simulink model "ccc_core"  (Simulink 7.4)
settings: Solver=ode45  StartTime=0.0  StopTime=10000  RelTol=1e-3
libraries: xbsIndex_r4 x236, cfa_library x64, casper_library_misc x7
(part 1 of 5)
settings Model: Creator=Administrator  LastModifiedBy=rprimian
settings OptimizationCC: InitFltsAndDblsToZero=on

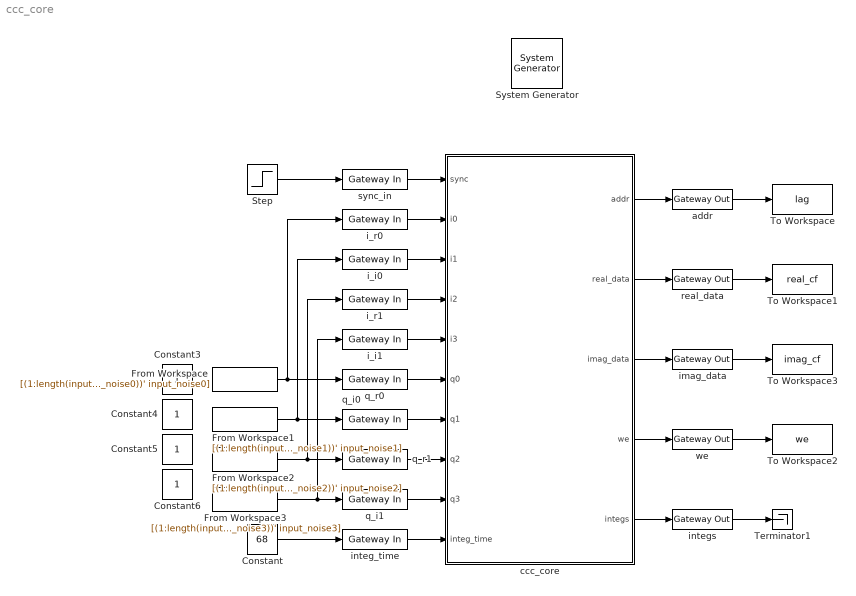
== system ccc_core ==
  " System Generator" : xbsIndex_r4/ System Generator  Tag=genX  SystemSampleTime=-1  xilinxfamily=virtex2p  part=xc2vp50  speed=-7  package=ff1152  synthesis_tool=XST  clock_wrapper=Clock Enables  directory=./correlator_core  testbench=off  simulink_period=1  sysclk_period=100  dcm_input_clock_period=100  incr_netlist=off  trim_vbits=Everywhere in SubSystem  dbl_ovrd=According to Block Masks  core_generation=According to Block Masks  run_coregen=off  deprecated_control=off  eval_field=0  block_type=sysgen
      settings: block_version=10.1.3
  Constant : Constant  Value=68  OutDataType=sfix(16)  OutScaling=2^0
  Constant{3..6} (4 alike) : Constant  OutDataType=sfix(16)  OutScaling=2^0
  From Workspace : FromWorkspace  VariableName=[(1:length(input_noise0))' input_noise0]  SampleTime=1  Interpolate=off  OutputAfterFinalValue=Setting to zero
  From Workspace1 : FromWorkspace  VariableName=[(1:length(input_noise1))' input_noise1]  SampleTime=1  Interpolate=off  OutputAfterFinalValue=Setting to zero
  From Workspace2 : FromWorkspace  VariableName=[(1:length(input_noise2))' input_noise2]  SampleTime=1  Interpolate=off  OutputAfterFinalValue=Setting to zero
  From Workspace3 : FromWorkspace  VariableName=[(1:length(input_noise3))' input_noise3]  SampleTime=1  Interpolate=off  OutputAfterFinalValue=Setting to zero
  Step : Step  Time=100  SampleTime=0
  Terminator1 : Terminator
  To Workspace : ToWorkspace  VariableName=lag  SampleTime=-1  SaveFormat=Array
  To Workspace1 : ToWorkspace  VariableName=real_cf  SampleTime=-1  SaveFormat=Array
  To Workspace2 : ToWorkspace  VariableName=we  SampleTime=-1  SaveFormat=Array
  To Workspace3 : ToWorkspace  VariableName=imag_cf  SampleTime=-1  SaveFormat=Array
  addr : xbsIndex_r4/Gateway Out  hdl_port=on  timing_constraint=None  locs_specified=off  LOCs={}  block_type=gatewayout
      settings: infoedit="Gateway out block.  Converts Xilinx fixed point inputs into ouputs of type Simulink integer, double, or fixed point.<P><P>Hardware notes:  In hardware these blocks become top level output ports or are discarded, depending on how they are configured."  block_version=10.1.3
  ccc_core : Subsystem
  i_i0 : xbsIndex_r4/Gateway In  arith_type=Unsigned  n_bits=2  bin_pt=0  quantization=Truncate  overflow=Wrap  period=1  dbl_ovrd=off  timing_constraint=None  locs_specified=off  LOCs={}  hdl_port=on  block_type=gatewayin
      settings: infoedit="Gateway in block.  Converts inputs of type Simulink integer, double and fixed point to  Xilinx fixed point type.<br><br>Hardware notes:  In hardware these blocks become top level input ports."  block_version=10.1.3
  i_i1 : xbsIndex_r4/Gateway In  arith_type=Unsigned  n_bits=2  bin_pt=0  quantization=Truncate  overflow=Wrap  period=1  dbl_ovrd=off  timing_constraint=None  locs_specified=off  LOCs={}  hdl_port=on  block_type=gatewayin
      settings: infoedit="Gateway in block.  Converts inputs of type Simulink integer, double and fixed point to  Xilinx fixed point type.<br><br>Hardware notes:  In hardware these blocks become top level input ports."  block_version=10.1.3
  i_r0 : xbsIndex_r4/Gateway In  arith_type=Unsigned  n_bits=2  bin_pt=0  quantization=Truncate  overflow=Flag as error  period=1  dbl_ovrd=off  timing_constraint=None  locs_specified=off  LOCs={}  hdl_port=on  block_type=gatewayin
      settings: infoedit="Gateway in block.  Converts inputs of type Simulink integer, double and fixed point to  Xilinx fixed point type.<br><br>Hardware notes:  In hardware these blocks become top level input ports."  block_version=10.1.3
  i_r1 : xbsIndex_r4/Gateway In  arith_type=Unsigned  n_bits=2  bin_pt=0  quantization=Truncate  overflow=Wrap  period=1  dbl_ovrd=off  timing_constraint=None  locs_specified=off  LOCs={}  hdl_port=on  block_type=gatewayin
      settings: infoedit="Gateway in block.  Converts inputs of type Simulink integer, double and fixed point to  Xilinx fixed point type.<br><br>Hardware notes:  In hardware these blocks become top level input ports."  block_version=10.1.3
  imag_data : xbsIndex_r4/Gateway Out  hdl_port=on  timing_constraint=None  locs_specified=off  LOCs={}  block_type=gatewayout
      settings: infoedit="Gateway out block.  Converts Xilinx fixed point inputs into ouputs of type Simulink integer, double, or fixed point.<P><P>Hardware notes:  In hardware these blocks become top level output ports or are discarded, depending on how they are configured."  block_version=10.1.3
  integ_time : xbsIndex_r4/Gateway In  arith_type=Unsigned  n_bits=32  bin_pt=0  quantization=Truncate  overflow=Wrap  period=1  dbl_ovrd=off  timing_constraint=None  locs_specified=off  LOCs={}  hdl_port=on  block_type=gatewayin
      settings: infoedit="Gateway in block.  Converts inputs of type Simulink integer, double and fixed point to  Xilinx fixed point type.<P><P>Hardware notes:  In hardware these blocks become top level input ports."  block_version=10.1.3
  integs : xbsIndex_r4/Gateway Out  hdl_port=on  timing_constraint=None  locs_specified=off  LOCs={}  block_type=gatewayout
      settings: infoedit="Gateway out block.  Converts Xilinx fixed point inputs into ouputs of type Simulink integer, double, or fixed point.<P><P>Hardware notes:  In hardware these blocks become top level output ports or are discarded, depending on how they are configured."  block_version=10.1.3
  q_i0 : xbsIndex_r4/Gateway In  arith_type=Unsigned  n_bits=2  bin_pt=0  quantization=Truncate  overflow=Wrap  period=1  dbl_ovrd=off  timing_constraint=None  locs_specified=off  LOCs={}  hdl_port=on  block_type=gatewayin
      settings: infoedit="Gateway in block.  Converts inputs of type Simulink integer, double and fixed point to  Xilinx fixed point type.<br><br>Hardware notes:  In hardware these blocks become top level input ports."  block_version=10.1.3
  q_i1 : xbsIndex_r4/Gateway In  arith_type=Unsigned  n_bits=2  bin_pt=0  quantization=Truncate  overflow=Wrap  period=1  dbl_ovrd=off  timing_constraint=None  locs_specified=off  LOCs={}  hdl_port=on  block_type=gatewayin
      settings: infoedit="Gateway in block.  Converts inputs of type Simulink integer, double and fixed point to  Xilinx fixed point type.<br><br>Hardware notes:  In hardware these blocks become top level input ports."  block_version=10.1.3
  q_r0 : xbsIndex_r4/Gateway In  arith_type=Unsigned  n_bits=2  bin_pt=0  quantization=Truncate  overflow=Wrap  period=1  dbl_ovrd=off  timing_constraint=None  locs_specified=off  LOCs={}  hdl_port=on  block_type=gatewayin
      settings: infoedit="Gateway in block.  Converts inputs of type Simulink integer, double and fixed point to  Xilinx fixed point type.<br><br>Hardware notes:  In hardware these blocks become top level input ports."  block_version=10.1.3
  q_r1 : xbsIndex_r4/Gateway In  arith_type=Unsigned  n_bits=2  bin_pt=0  quantization=Truncate  overflow=Wrap  period=1  dbl_ovrd=off  timing_constraint=None  locs_specified=off  LOCs={}  hdl_port=on  block_type=gatewayin
      settings: infoedit="Gateway in block.  Converts inputs of type Simulink integer, double and fixed point to  Xilinx fixed point type.<br><br>Hardware notes:  In hardware these blocks become top level input ports."  block_version=10.1.3
  real_data : xbsIndex_r4/Gateway Out  hdl_port=on  timing_constraint=None  locs_specified=off  LOCs={}  block_type=gatewayout
      settings: infoedit="Gateway out block.  Converts Xilinx fixed point inputs into ouputs of type Simulink integer, double, or fixed point.<P><P>Hardware notes:  In hardware these blocks become top level output ports or are discarded, depending on how they are configured."  block_version=10.1.3
  sync_in : xbsIndex_r4/Gateway In  arith_type=Boolean  n_bits=16  bin_pt=14  quantization="Round  (unbiased: +/- Inf)"  overflow=Saturate  period=1  dbl_ovrd=off  timing_constraint=None  locs_specified=off  LOCs={}  hdl_port=on  block_type=gatewayin
      settings: infoedit="Gateway in block.  Converts inputs of type Simulink integer, double and fixed point to  Xilinx fixed point type.<P><P>Hardware notes:  In hardware these blocks become top level input ports."  block_version=10.1.3
  we : xbsIndex_r4/Gateway Out  hdl_port=on  timing_constraint=None  locs_specified=off  LOCs={}  block_type=gatewayout
      settings: infoedit="Gateway out block.  Converts Xilinx fixed point inputs into ouputs of type Simulink integer, double, or fixed point.<P><P>Hardware notes:  In hardware these blocks become top level output ports or are discarded, depending on how they are configured."  block_version=10.1.3
  wires:
  sync_in/1 -> ccc_core/1(sync)
  i_r0/1 -> ccc_core/2(i0)
  i_i0/1 -> ccc_core/3(i1)
  i_r1/1 -> ccc_core/4(i2)
  i_i1/1 -> ccc_core/5(i3)
  q_r0/1 -> ccc_core/6(q0)
  q_i0/1 -> ccc_core/7(q1)
  q_r1/1 -> ccc_core/8(q2)
  q_i1/1 -> ccc_core/9(q3)
  Step/1 -> sync_in/1
  integ_time/1 -> ccc_core/10(integ_time)
  Constant/1 -> integ_time/1
  addr/1 -> To Workspace/1
  real_data/1 -> To Workspace1/1
  we/1 -> To Workspace2/1
  From Workspace/1 -> i_r0/1, q_r0/1
  From Workspace1/1 -> i_i0/1, q_i0/1
  From Workspace2/1 -> i_r1/1, q_r1/1
  From Workspace3/1 -> i_i1/1, q_i1/1
  ccc_core/1(addr) -> addr/1
  ccc_core/2(real_data) -> real_data/1
  imag_data/1 -> To Workspace3/1
  ccc_core/3(imag_data) -> imag_data/1
  ccc_core/4(we) -> we/1
  ccc_core/5(integs) -> integs/1
  integs/1 -> Terminator1/1

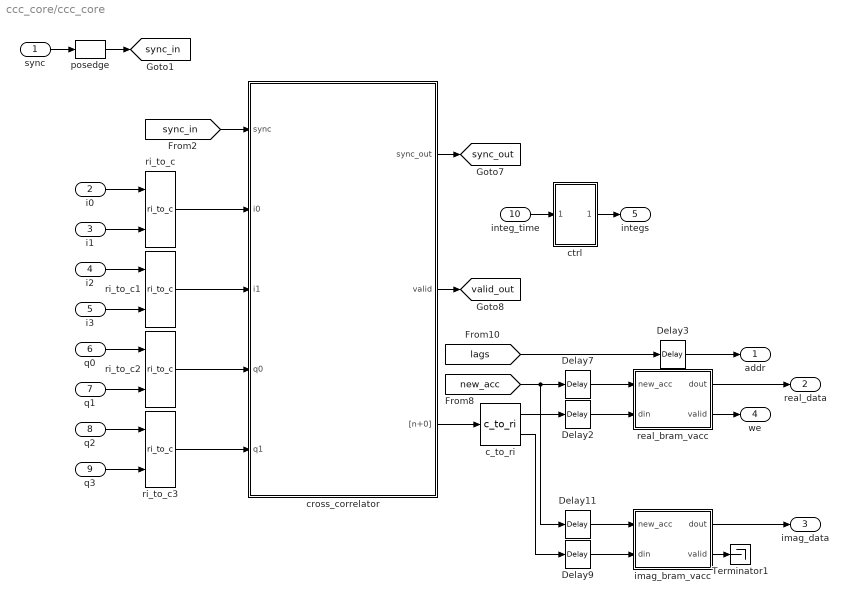
== system ccc_core/ccc_core ==
  sync : Inport
  i0 : Inport  Port=2
  i1 : Inport  Port=3
  i2 : Inport  Port=4
  i3 : Inport  Port=5
  q0 : Inport  Port=6
  q1 : Inport  Port=7
  q2 : Inport  Port=8
  q3 : Inport  Port=9
  integ_time : Inport  Port=10
  Delay{2,7,9,11} (4 alike) : xbsIndex_r4/Delay  en=off  latency=1  dbl_ovrd=off  reg_retiming=off  block_type=delay
      settings: block_version=11.4
  Delay3 : xbsIndex_r4/Delay  en=off  latency=0  dbl_ovrd=off  reg_retiming=off  block_type=delay
      settings: block_version=11.4
  Terminator1 : Terminator
  c_to_ri : casper_library_misc/c_to_ri  SystemSampleTime=-1  n_bits=11  bin_pt=0
      settings: AttributesFormatString=11_0 r/i
  cross_correlator : Subsystem  AncestorBlock=cfa_library/cross_correlator  mask(cross_correlator){total_lags=4, n_inputs=1, use_2bit=on, complex_in=on, input_bit_width=8, input_bin_pt=7, specify_data_type=off, output_bit_width=16, output_bin_pt=14, quantization=Truncate, overflow=Wrap, specify_mult=off, mult_spec=Behavioral, specify_add=off, add_spec=Fabric, mult_delay=3, add_delay=2, overall_delay=2, single_output=on}
      mask prompts: total_lags "Total Lags Centered at Zero: (2^?)"; n_inputs "Number of Simultaneous Inputs: (2^?)"; use_2bit "Use special 2-bit binary encoding"; complex_in "Complex inputs"; input_bit_width "Input Bit Width:"; input_bin_pt "Input Binary Point:"; specify_data_type "Specify output data type"; output_bit_width "Output Bit Width:"; output_bin_pt "Output Binary Point:"; quantization "Quantization Behavior:"; overflow "Overflow Behavior"; specify_mult "Specify multiplier use (behavioural HDL if not specified)"; mult_spec "Multiplier specification:"; specify_add "Specify adder use (behavioural HDL if not specified)"; add_spec "Adder specification:"; mult_delay "Mult Latency:"; add_delay "Add Latency:"; overall_delay "Overall latency:"; single_output "Provide single output stream"
      mask help: This time-domain cross correlator accepts two real time-series and outputs the cross-correlation function for the given set of lags. The output is accumulated so that for every two input samples there is exactly one output sample.
      mask init:
      | cross_correlator_init(gcb,...
      |     'total_lags', total_lags,...
      |     'n_inputs', n_inputs,...
      |     'use_2bit', use_2bit,...
      |     'input_bit_width', input_bit_width,...
      |     'input_bin_pt', input_bin_pt,...
      |     'complex_in', complex_in,...
      |     'specify_data_type', specify_data_type,...
      |     'output_bit_width', output_bit_width,...
      |     'output_bin_pt', output_bin_pt,...
      |     'quantization', quantization,...
      |     'overflow', overflow,...
      |     'specify_mult', specify_mult,...
      |     'mult_spec', mult_spec,...
      |     'specify_add', specify_add,...
      |     'add_spec', add_spec,...
      |     'mult_delay', mult_delay,...
      |     'add_delay', add_delay,...
      |     'overall_delay', overall_delay,...
      |     'single_output', single_output);
      settings: AttributesFormatString=|
      | 16 lags, Demux: 2, Outputs: 1
      | Special 2-bit complex binary encoding
      |  Mult: Behavioral, Add: Fabric
      mask StyleString: edit,edit,checkbox,checkbox,edit,edit,checkbox,edit,edit,popup(Truncate|Round (unbiased: +/- Inf)|Round (unbiased: Even Values)),popup(Wrap|Saturate|Flag as error),checkbox,popup(Behavioral|Core|Embedded),checkbox,popup(Fabric|DSP48),edit,edit,edit,checkbox
      mask CallbackString:
      | ||use_2bit = get_param(gcb,'use_2bit');
      | enables = get_param(gcb, 'MaskEnables');
      | if( strcmp(use_2bit,'on')),
      |     enables{4} = 'on';
      |     enables{5} = 'off';
      |     enables{6} = 'off';
      | else
      |     enables{4} = 'off';
      |     enables{5} = 'on';
      |     enables{6} = 'on';
      | end
      | set_param(gcb, 'MaskEnables', enables);
      | ||||specify_data_type = get_param(gcb,'specify_data_type');
      | enables = get_param(gcb, 'MaskEnables');
      | if( strcmp(specify_data_type,'off')),
      |     enables{8} = 'off';
      |     enables{9} = 'off';
      |     enables{10} = 'off';
      |     enables{11} = 'off';
      | else
      |     enables{8} = 'on';
      |     enables{9} = 'on';
      |     enables{10} = 'on';
      |     enables{11} = 'on';
      | end
      | set_param(gcb, 'MaskEnables', enables);
      | |||||specify_mult = get_param(gcb,'specify_mult');
      | enables = get_param(gcb, 'MaskEnables');
      | if( strcmp(specify_mult,'off')),
      |     enables{13} = 'off';
      | else
      |     enables{13} = 'on';
      | end
      | set_param(gcb, 'MaskEnables', enables);
      | ||specify_add = get_param(gcb,'specify_add');
      | enables = get_param(gcb, 'MaskEnables');
      | if( strcmp(specify_add,'off')),
      |     enables{15} = 'off';
      | else
      |     enables{15} = 'on';
      | end
      | set_param(gcb, 'MaskEnables', enables);
      | |||||
      mask TabNameString: Basic,Basic,Input,Input,Input,Input,Output,Output,Output,Output,Output,Implementation,Implementation,Implementation,Implementation,Implementation,Implementation,Implementation,Basic
  ctrl : Subsystem  mask{total_lags=4}
      mask prompts: total_lags "Total Lags (2^?):"
      mask Display: fprintf('CTRL');
  imag_bram_vacc : Subsystem  mask(simple_bram_vacc){vec_len=16, arith_type=Signed, n_bits=32, bin_pt=0, add_latency=3}
      mask prompts: vec_len "Vector length:"; arith_type "Output type:"; n_bits "Bit width (output):"; bin_pt "Binary point (output):"; add_latency "Adder latency:"
      mask help: This simple vector accumulator is based on a shift register. It outputs its previous accumulated vector after a new_acc pulse is received.
      mask init:
      | simple_bram_vacc_init(gcb, ...
      |     'vec_len', vec_len, ...
      |     'arith_type', arith_type, ...
      |     'n_bits', n_bits, ...
      |     'bin_pt', bin_pt);
      mask StyleString: edit,popup(Signed|Unsigned),edit,edit,edit
  posedge : casper_library_misc/posedge  Tag=Rising Edge Detector  SystemSampleTime=-1
  real_bram_vacc : Subsystem  mask(simple_bram_vacc){vec_len=16, arith_type=Signed, n_bits=32, bin_pt=0, add_latency=3}
      mask prompts: vec_len "Vector length:"; arith_type "Output type:"; n_bits "Bit width (output):"; bin_pt "Binary point (output):"; add_latency "Adder latency:"
      mask help: This simple vector accumulator is based on a shift register. It outputs its previous accumulated vector after a new_acc pulse is received.
      mask init:
      | simple_bram_vacc_init(gcb, ...
      |     'vec_len', vec_len, ...
      |     'arith_type', arith_type, ...
      |     'n_bits', n_bits, ...
      |     'bin_pt', bin_pt);
      mask StyleString: edit,popup(Signed|Unsigned),edit,edit,edit
  ri_to_c{,1..3} (4 alike) : casper_library_misc/ri_to_c  SystemSampleTime=-1
  addr : Outport
  real_data : Outport  Port=2
  imag_data : Outport  Port=3
  we : Outport  Port=4
  integs : Outport  Port=5
  tag scope: sync_in=global, sync_out=global, valid_out=global
  wires:
  Delay2/1 -> real_bram_vacc/2(din)
  [lags] -> Delay3/1
  [new_acc] -> Delay7/1, Delay11/1
  real_bram_vacc/1(dout) -> real_data/1
  sync/1 -> posedge/1
  Delay3/1 -> addr/1
  real_bram_vacc/2(valid) -> we/1
  integ_time/1 -> ctrl/1(integ_time)
  ctrl/1(integs) -> integs/1
  posedge/1 -> [sync_in]
  cross_correlator/1(sync_out) -> [sync_out]
  cross_correlator/2(valid) -> [valid_out]
  [sync_in] -> cross_correlator/1(sync)
  Delay7/1 -> real_bram_vacc/1(new_acc)
  ri_to_c2/1 -> cross_correlator/4(q0)
  ri_to_c3/1 -> cross_correlator/5(q1)
  c_to_ri/1 -> Delay2/1
  cross_correlator/3("[n+0]") -> c_to_ri/1
  Delay9/1 -> imag_bram_vacc/2(din)
  imag_bram_vacc/1(dout) -> imag_data/1
  Delay11/1 -> imag_bram_vacc/1(new_acc)
  c_to_ri/2 -> Delay9/1
  imag_bram_vacc/2(valid) -> Terminator1/1
  ri_to_c/1 -> cross_correlator/2(i0)
  ri_to_c1/1 -> cross_correlator/3(i1)
  i0/1 -> ri_to_c/1
  i1/1 -> ri_to_c/2
  i2/1 -> ri_to_c1/1
  i3/1 -> ri_to_c1/2
  q0/1 -> ri_to_c2/1
  q1/1 -> ri_to_c2/2
  q2/1 -> ri_to_c3/1
  q3/1 -> ri_to_c3/2
